simulink model "CM340A_AdcDiagc"  (R2013b)
settings: Solver=FixedStepDiscrete  SolverMode=SingleTasking  StartTime=0.0  StopTime=1  FixedStep=0.002  RelTol=1e-3
values from neighbouring files (symbols this model uses):
  Adc0Diagc = DataDict.NTC    [CM340A_AdcDiagc_DataDict.m]
  Adc1Diagc = DataDict.NTC    [CM340A_AdcDiagc_DataDict.m]
  ADCDIAG0REFVOLT_VOLT_F32 = DataDict.Constant    [CM340A_AdcDiagc_DataDict.m]
  ADCDIAG2REFVOLT_VOLT_F32 = DataDict.Constant    [CM340A_AdcDiagc_DataDict.m]
  ADCDIAG4REFVOLT_VOLT_F32 = DataDict.Constant    [CM340A_AdcDiagc_DataDict.m]
  AdcDiagcNtc0x032FailStep = DataDict.Calibration    [CM340A_AdcDiagc_DataDict.m]
  AdcDiagcNtc0x032PassStep = DataDict.Calibration    [CM340A_AdcDiagc_DataDict.m]
  AdcDiagcNtc0x033FailStep = DataDict.Calibration    [CM340A_AdcDiagc_DataDict.m]
  AdcDiagcNtc0x033PassStep = DataDict.Calibration    [CM340A_AdcDiagc_DataDict.m]
  AdcDiagcSt = DataDict.PIM    [CM340A_AdcDiagc_DataDict.m]
  ADCDIAGPARFLTPRM_CNT_U08 = DataDict.Constant    [CM340A_AdcDiagc_DataDict.m]
  ADCDIAGSCANGROUP2REFFLTPRM_CNT_U08 = DataDict.Constant    [CM340A_AdcDiagc_DataDict.m]
  ADCDIAGSCANGROUP3REFFLTPRM_CNT_U08 = DataDict.Constant    [CM340A_AdcDiagc_DataDict.m]
  ADCDIAGSCANGROUPENDREFVOLT_VOLT_F32 = DataDict.Constant    [CM340A_AdcDiagc_DataDict.m]
  ADCDIAGSCANGROUPSTRTREFVOLT_VOLT_F32 = DataDict.Constant    [CM340A_AdcDiagc_DataDict.m]
  ADCDNECRPARERRCLR_CNT_U08 = DataDict.Constant    [CM340A_AdcDiagc_DataDict.m]
  ADCDNPERPARERRMASK_CNT_U08 = DataDict.Constant    [CM340A_AdcDiagc_DataDict.m]
  VIRTCH21_CNT_U08 = DataDict.Constant    [CM340A_AdcDiagc_DataDict.m]
  VIRTCH22_CNT_U08 = DataDict.Constant    [CM340A_AdcDiagc_DataDict.m]
  VIRTCH23_CNT_U08 = DataDict.Constant    [CM340A_AdcDiagc_DataDict.m]
undefined symbols (not defined in the file or in its folder): NtcSts1, sigbuilder_block, SigQlfr1
libraries: simulink x42, CM340A_AdcDiagc_Library x40
(part 4 of 4)

== system CM340A_AdcDiagc/AdcDiagc/AdcDiagcPer1/NTC Fault Processing1/SetNtcSts/Enabled Subsystem ==
  In1 : Inport
  Enable : EnablePort
  Bitwise Operator : simulink/Logic and Bit Operations/Bitwise Operator  logicop=OR  UseBitMask=off  NumInputPorts=2  BitMask=bin2dec('11011001')  BitMaskRealWorld=Stored Integer
  CopyRight2 : Subsystem  Description=|  mask(Copyright Information){none=on}
      | Copyright info block.                                               
      |                                                                     
      | Place copyright information at the top of every subsystem in design.
      mask prompts: none "No parameters"
      mask help: Place copyright information at the top of every subsystem in design.
      mask Display:
      | NxtrConf = 'Nexteer Confidential';
      | 
      | sys = bdroot; %handle for the current model ("system")
      | first = get_param(sys,'Created');
      | first = first(end-3:end);  %year is last four digits
      | 
      | last = get_param(sys,'LastModifiedDate');
      | if isempty(last)
      |     last = datestr(now,'yyyy');
      | else
      |     last = last(end-3:end);
      | end
      | 
      | if strcmp(first,last)
      |     fprintf('%s -- Copyright %s Nexteer',NxtrConf,first)
      | else
      |     fprintf('%s -- %s%s- %s Nexteer',NxtrConf,char(169),first,last)
      | end
  Data Store Read : DataStoreRead  DataStoreName=Adc1DynDiagcPrm
  Data Store Write1 : DataStoreWrite  DataStoreName=Adc1DynDiagcPrm
  wires:
  In1/1 -> Bitwise Operator/1
  Bitwise Operator/1 -> Data Store Write1/1
  Data Store Read/1 -> Bitwise Operator/2

== system CM340A_AdcDiagc/AdcDiagc/AdcDiagcPer1/Adc Daigc Pointer/Strt & End Ptr Store/State 0/CopyRight2 ==

== system CM340A_AdcDiagc/AdcDiagc/AdcDiagcPer1/Adc Daigc Pointer/Strt & End Ptr Store/State 1/CopyRight2 ==

== system CM340A_AdcDiagc/AdcDiagc/AdcDiagcPer1/Adc Daigc Pointer/Strt & End Ptr Store/State 2/CopyRight2 ==

== system CM340A_AdcDiagc/AdcDiagc/AdcDiagcPer1/Adc Daigc Pointer/Strt & End Ptr Store/State 4/CopyRight2 ==

== system CM340A_AdcDiagc/AdcDiagc/AdcDiagcPer1/Adc Daigc Pointer/Strt & End Ptr Store/State 6/CopyRight2 ==

== system CM340A_AdcDiagc/AdcDiagc/AdcDiagcPer1/Adc0 Diagc/Adc0 Scan Group Strt and End Ref Voltage Diagc/Subsystem/CopyRight2 ==

== system CM340A_AdcDiagc/AdcDiagc/AdcDiagcPer1/Adc0 Diagc/Adc0 Scan Group Strt and End Ref Voltage Diagc/Subsystem1/CopyRight2 ==

== system CM340A_AdcDiagc/AdcDiagc/AdcDiagcPer1/Adc0 Diagc/State 0, 2, 4, 6/State 0/CopyRight2 ==

== system CM340A_AdcDiagc/AdcDiagc/AdcDiagcPer1/Adc0 Diagc/State 0, 2, 4, 6/State 0/Subsystem ==
  Parameter Byte : Inport
  FltCntrPrev : Inport  Port=2
  Add : Sum
  Bitwise Operator : simulink/Logic and Bit Operations/Bitwise Operator  logicop=AND  UseBitMask=off  NumInputPorts=2  BitMask=bin2dec('01111111')  BitMaskRealWorld=Stored Integer
  Constant : Constant  Value=0
  Constant1 : Constant  Value=127  OutDataTypeStr=uint8
  CopyRight2 : Subsystem  Description=|  mask(Copyright Information){none=on}
      | Copyright info block.                                               
      |                                                                     
      | Place copyright information at the top of every subsystem in design.
      mask prompts: none "No parameters"
      mask help: Place copyright information at the top of every subsystem in design.
      mask Display:
      | NxtrConf = 'Nexteer Confidential';
      | 
      | sys = bdroot; %handle for the current model ("system")
      | first = get_param(sys,'Created');
      | first = first(end-3:end);  %year is last four digits
      | 
      | last = get_param(sys,'LastModifiedDate');
      | if isempty(last)
      |     last = datestr(now,'yyyy');
      | else
      |     last = last(end-3:end);
      | end
      | 
      | if strcmp(first,last)
      |     fprintf('%s -- Copyright %s Nexteer',NxtrConf,first)
      | else
      |     fprintf('%s -- %s%s- %s Nexteer',NxtrConf,char(169),first,last)
      | end
  Data Type Conversion2 : DataTypeConversion  OutDataTypeStr=uint8
  Relational Operator : RelationalOperator  Operator=>  OutDataTypeStr=boolean
  Scope1 : Scope  NumInputPorts=2
      settings: ShowLegends=on  TimeRange=1000  YMin=-2~0  YMax=2~256  SaveName=ScopeData3
  FltCntr : Outport
  wires:
  Constant/1 -> Relational Operator/2
  Parameter Byte/1 -> Scope1/1, Relational Operator/1
  Relational Operator/1 -> Data Type Conversion2/1
  Add/1 -> Bitwise Operator/1
  Bitwise Operator/1 -> FltCntr/1, Scope1/2
  FltCntrPrev/1 -> Add/2
  Data Type Conversion2/1 -> Add/1
  Constant1/1 -> Bitwise Operator/2

== system CM340A_AdcDiagc/AdcDiagc/AdcDiagcPer1/Adc0 Diagc/State 0, 2, 4, 6/State 2/CopyRight2 ==

== system CM340A_AdcDiagc/AdcDiagc/AdcDiagcPer1/Adc0 Diagc/State 0, 2, 4, 6/State 2/Subsystem1 ==
  Parameter Byte : Inport
  FltCntrPrev : Inport  Port=2
  Add : Sum
  Bitwise Operator : simulink/Logic and Bit Operations/Bitwise Operator  logicop=AND  UseBitMask=off  NumInputPorts=2  BitMask=bin2dec('01111111')  BitMaskRealWorld=Stored Integer
  Constant : Constant  Value=0
  Constant1 : Constant  Value=127  OutDataTypeStr=uint8
  CopyRight2 : Subsystem  Description=|  mask(Copyright Information){none=on}
      | Copyright info block.                                               
      |                                                                     
      | Place copyright information at the top of every subsystem in design.
      mask prompts: none "No parameters"
      mask help: Place copyright information at the top of every subsystem in design.
      mask Display:
      | NxtrConf = 'Nexteer Confidential';
      | 
      | sys = bdroot; %handle for the current model ("system")
      | first = get_param(sys,'Created');
      | first = first(end-3:end);  %year is last four digits
      | 
      | last = get_param(sys,'LastModifiedDate');
      | if isempty(last)
      |     last = datestr(now,'yyyy');
      | else
      |     last = last(end-3:end);
      | end
      | 
      | if strcmp(first,last)
      |     fprintf('%s -- Copyright %s Nexteer',NxtrConf,first)
      | else
      |     fprintf('%s -- %s%s- %s Nexteer',NxtrConf,char(169),first,last)
      | end
  Data Type Conversion2 : DataTypeConversion  OutDataTypeStr=uint8
  Relational Operator : RelationalOperator  Operator=>  OutDataTypeStr=boolean
  Scope1 : Scope  NumInputPorts=2
      settings: ShowLegends=on  TimeRange=1000  YMin=-2~0  YMax=2~256  SaveName=ScopeData3
  FltCntr : Outport
  wires:
  Constant/1 -> Relational Operator/2
  Parameter Byte/1 -> Scope1/1, Relational Operator/1
  Relational Operator/1 -> Data Type Conversion2/1
  Add/1 -> Bitwise Operator/1
  Bitwise Operator/1 -> FltCntr/1, Scope1/2
  FltCntrPrev/1 -> Add/2
  Data Type Conversion2/1 -> Add/1
  Constant1/1 -> Bitwise Operator/2

== system CM340A_AdcDiagc/AdcDiagc/AdcDiagcPer1/Adc0 Diagc/State 0, 2, 4, 6/State 4/CopyRight2 ==

== system CM340A_AdcDiagc/AdcDiagc/AdcDiagcPer1/Adc0 Diagc/State 0, 2, 4, 6/State 4/Subsystem ==
  Parameter Byte : Inport
  FltCntrPrev : Inport  Port=2
  Add : Sum
  Bitwise Operator : simulink/Logic and Bit Operations/Bitwise Operator  logicop=AND  UseBitMask=off  NumInputPorts=2  BitMask=bin2dec('01111111')  BitMaskRealWorld=Stored Integer
  Constant : Constant  Value=0
  Constant1 : Constant  Value=127  OutDataTypeStr=uint8
  CopyRight2 : Subsystem  Description=|  mask(Copyright Information){none=on}
      | Copyright info block.                                               
      |                                                                     
      | Place copyright information at the top of every subsystem in design.
      mask prompts: none "No parameters"
      mask help: Place copyright information at the top of every subsystem in design.
      mask Display:
      | NxtrConf = 'Nexteer Confidential';
      | 
      | sys = bdroot; %handle for the current model ("system")
      | first = get_param(sys,'Created');
      | first = first(end-3:end);  %year is last four digits
      | 
      | last = get_param(sys,'LastModifiedDate');
      | if isempty(last)
      |     last = datestr(now,'yyyy');
      | else
      |     last = last(end-3:end);
      | end
      | 
      | if strcmp(first,last)
      |     fprintf('%s -- Copyright %s Nexteer',NxtrConf,first)
      | else
      |     fprintf('%s -- %s%s- %s Nexteer',NxtrConf,char(169),first,last)
      | end
  Data Type Conversion2 : DataTypeConversion  OutDataTypeStr=uint8
  Relational Operator : RelationalOperator  Operator=>  OutDataTypeStr=boolean
  Scope1 : Scope  NumInputPorts=2
      settings: ShowLegends=on  TimeRange=1000  YMin=-2~0  YMax=2~256  SaveName=ScopeData3
  FltCntr : Outport
  wires:
  Constant/1 -> Relational Operator/2
  Parameter Byte/1 -> Scope1/1, Relational Operator/1
  Relational Operator/1 -> Data Type Conversion2/1
  Add/1 -> Bitwise Operator/1
  Bitwise Operator/1 -> FltCntr/1, Scope1/2
  FltCntrPrev/1 -> Add/2
  Data Type Conversion2/1 -> Add/1
  Constant1/1 -> Bitwise Operator/2

== system CM340A_AdcDiagc/AdcDiagc/AdcDiagcPer1/Adc0 Diagc/State 0, 2, 4, 6/State 6/CopyRight2 ==

== system CM340A_AdcDiagc/AdcDiagc/AdcDiagcPer1/Adc0 Diagc/State 0, 2, 4, 6/State 6/Subsystem ==
  Parameter Byte : Inport
  FltCntrPrev : Inport  Port=2
  Add : Sum
  Bitwise Operator : simulink/Logic and Bit Operations/Bitwise Operator  logicop=AND  UseBitMask=off  NumInputPorts=2  BitMask=bin2dec('01111111')  BitMaskRealWorld=Stored Integer
  Constant : Constant  Value=0
  Constant1 : Constant  Value=127  OutDataTypeStr=uint8
  CopyRight2 : Subsystem  Description=|  mask(Copyright Information){none=on}
      | Copyright info block.                                               
      |                                                                     
      | Place copyright information at the top of every subsystem in design.
      mask prompts: none "No parameters"
      mask help: Place copyright information at the top of every subsystem in design.
      mask Display:
      | NxtrConf = 'Nexteer Confidential';
      | 
      | sys = bdroot; %handle for the current model ("system")
      | first = get_param(sys,'Created');
      | first = first(end-3:end);  %year is last four digits
      | 
      | last = get_param(sys,'LastModifiedDate');
      | if isempty(last)
      |     last = datestr(now,'yyyy');
      | else
      |     last = last(end-3:end);
      | end
      | 
      | if strcmp(first,last)
      |     fprintf('%s -- Copyright %s Nexteer',NxtrConf,first)
      | else
      |     fprintf('%s -- %s%s- %s Nexteer',NxtrConf,char(169),first,last)
      | end
  Data Type Conversion2 : DataTypeConversion  OutDataTypeStr=uint8
  Relational Operator : RelationalOperator  Operator=>  OutDataTypeStr=boolean
  Scope1 : Scope  NumInputPorts=2
      settings: ShowLegends=on  TimeRange=1000  YMin=-2~0  YMax=2~256  SaveName=ScopeData3
  FltCntr : Outport
  wires:
  Constant/1 -> Relational Operator/2
  Parameter Byte/1 -> Scope1/1, Relational Operator/1
  Relational Operator/1 -> Data Type Conversion2/1
  Add/1 -> Bitwise Operator/1
  Bitwise Operator/1 -> FltCntr/1, Scope1/2
  FltCntrPrev/1 -> Add/2
  Data Type Conversion2/1 -> Add/1
  Constant1/1 -> Bitwise Operator/2

== system CM340A_AdcDiagc/AdcDiagc/AdcDiagcPer1/Adc1 Diagc/Adc1 Scan Group Strt and End Ref Voltage Diagc/Subsystem/CopyRight2 ==

== system CM340A_AdcDiagc/AdcDiagc/AdcDiagcPer1/Adc1 Diagc/Adc1 Scan Group Strt and End Ref Voltage Diagc/Subsystem1/CopyRight2 ==

== system CM340A_AdcDiagc/AdcDiagc/AdcDiagcPer1/Adc1 Diagc/State 0,2,4,6/State 0/CopyRight2 ==

== system CM340A_AdcDiagc/AdcDiagc/AdcDiagcPer1/Adc1 Diagc/State 0,2,4,6/State 0/Subsystem ==
  Parameter Byte : Inport
  FltCntrPrev : Inport  Port=2
  Add : Sum
  Bitwise Operator : simulink/Logic and Bit Operations/Bitwise Operator  logicop=AND  UseBitMask=off  NumInputPorts=2  BitMask=bin2dec('01111111')  BitMaskRealWorld=Stored Integer
  Constant : Constant  Value=0
  Constant1 : Constant  Value=127  OutDataTypeStr=uint8
  CopyRight2 : Subsystem  Description=|  mask(Copyright Information){none=on}
      | Copyright info block.                                               
      |                                                                     
      | Place copyright information at the top of every subsystem in design.
      mask prompts: none "No parameters"
      mask help: Place copyright information at the top of every subsystem in design.
      mask Display:
      | NxtrConf = 'Nexteer Confidential';
      | 
      | sys = bdroot; %handle for the current model ("system")
      | first = get_param(sys,'Created');
      | first = first(end-3:end);  %year is last four digits
      | 
      | last = get_param(sys,'LastModifiedDate');
      | if isempty(last)
      |     last = datestr(now,'yyyy');
      | else
      |     last = last(end-3:end);
      | end
      | 
      | if strcmp(first,last)
      |     fprintf('%s -- Copyright %s Nexteer',NxtrConf,first)
      | else
      |     fprintf('%s -- %s%s- %s Nexteer',NxtrConf,char(169),first,last)
      | end
  Data Type Conversion2 : DataTypeConversion  OutDataTypeStr=uint8
  Relational Operator : RelationalOperator  Operator=>  OutDataTypeStr=boolean
  Scope1 : Scope  NumInputPorts=2
      settings: ShowLegends=on  TimeRange=1000  YMin=-2~0  YMax=2~256  SaveName=ScopeData3
  FltCntr : Outport
  wires:
  Constant/1 -> Relational Operator/2
  Parameter Byte/1 -> Scope1/1, Relational Operator/1
  Relational Operator/1 -> Data Type Conversion2/1
  Add/1 -> Bitwise Operator/1
  Bitwise Operator/1 -> FltCntr/1, Scope1/2
  FltCntrPrev/1 -> Add/2
  Data Type Conversion2/1 -> Add/1
  Constant1/1 -> Bitwise Operator/2

== system CM340A_AdcDiagc/AdcDiagc/AdcDiagcPer1/Adc1 Diagc/State 0,2,4,6/State 2/CopyRight2 ==

== system CM340A_AdcDiagc/AdcDiagc/AdcDiagcPer1/Adc1 Diagc/State 0,2,4,6/State 2/Subsystem ==
  Parameter Byte : Inport
  FltCntrPrev : Inport  Port=2
  Add : Sum
  Bitwise Operator : simulink/Logic and Bit Operations/Bitwise Operator  logicop=AND  UseBitMask=off  NumInputPorts=2  BitMask=bin2dec('01111111')  BitMaskRealWorld=Stored Integer
  Constant : Constant  Value=0
  Constant1 : Constant  Value=127  OutDataTypeStr=uint8
  CopyRight2 : Subsystem  Description=|  mask(Copyright Information){none=on}
      | Copyright info block.                                               
      |                                                                     
      | Place copyright information at the top of every subsystem in design.
      mask prompts: none "No parameters"
      mask help: Place copyright information at the top of every subsystem in design.
      mask Display:
      | NxtrConf = 'Nexteer Confidential';
      | 
      | sys = bdroot; %handle for the current model ("system")
      | first = get_param(sys,'Created');
      | first = first(end-3:end);  %year is last four digits
      | 
      | last = get_param(sys,'LastModifiedDate');
      | if isempty(last)
      |     last = datestr(now,'yyyy');
      | else
      |     last = last(end-3:end);
      | end
      | 
      | if strcmp(first,last)
      |     fprintf('%s -- Copyright %s Nexteer',NxtrConf,first)
      | else
      |     fprintf('%s -- %s%s- %s Nexteer',NxtrConf,char(169),first,last)
      | end
  Data Type Conversion2 : DataTypeConversion  OutDataTypeStr=uint8
  Relational Operator : RelationalOperator  Operator=>  OutDataTypeStr=boolean
  Scope1 : Scope  NumInputPorts=2
      settings: ShowLegends=on  TimeRange=1000  YMin=-2~0  YMax=2~256  SaveName=ScopeData3
  FltCntr : Outport
  wires:
  Constant/1 -> Relational Operator/2
  Parameter Byte/1 -> Scope1/1, Relational Operator/1
  Relational Operator/1 -> Data Type Conversion2/1
  Add/1 -> Bitwise Operator/1
  Bitwise Operator/1 -> FltCntr/1, Scope1/2
  FltCntrPrev/1 -> Add/2
  Data Type Conversion2/1 -> Add/1
  Constant1/1 -> Bitwise Operator/2

== system CM340A_AdcDiagc/AdcDiagc/AdcDiagcPer1/Adc1 Diagc/State 0,2,4,6/State 4/CopyRight2 ==

== system CM340A_AdcDiagc/AdcDiagc/AdcDiagcPer1/Adc1 Diagc/State 0,2,4,6/State 4/Subsystem ==
  Parameter Byte : Inport
  FltCntrPrev : Inport  Port=2
  Add : Sum
  Bitwise Operator : simulink/Logic and Bit Operations/Bitwise Operator  logicop=AND  UseBitMask=off  NumInputPorts=2  BitMask=bin2dec('01111111')  BitMaskRealWorld=Stored Integer
  Constant : Constant  Value=0
  Constant1 : Constant  Value=127  OutDataTypeStr=uint8
  CopyRight2 : Subsystem  Description=|  mask(Copyright Information){none=on}
      | Copyright info block.                                               
      |                                                                     
      | Place copyright information at the top of every subsystem in design.
      mask prompts: none "No parameters"
      mask help: Place copyright information at the top of every subsystem in design.
      mask Display:
      | NxtrConf = 'Nexteer Confidential';
      | 
      | sys = bdroot; %handle for the current model ("system")
      | first = get_param(sys,'Created');
      | first = first(end-3:end);  %year is last four digits
      | 
      | last = get_param(sys,'LastModifiedDate');
      | if isempty(last)
      |     last = datestr(now,'yyyy');
      | else
      |     last = last(end-3:end);
      | end
      | 
      | if strcmp(first,last)
      |     fprintf('%s -- Copyright %s Nexteer',NxtrConf,first)
      | else
      |     fprintf('%s -- %s%s- %s Nexteer',NxtrConf,char(169),first,last)
      | end
  Data Type Conversion2 : DataTypeConversion  OutDataTypeStr=uint8
  Relational Operator : RelationalOperator  Operator=>  OutDataTypeStr=boolean
  Scope1 : Scope  NumInputPorts=2
      settings: ShowLegends=on  TimeRange=1000  YMin=-2~0  YMax=2~256  SaveName=ScopeData3
  FltCntr : Outport
  wires:
  Constant/1 -> Relational Operator/2
  Parameter Byte/1 -> Scope1/1, Relational Operator/1
  Relational Operator/1 -> Data Type Conversion2/1
  Add/1 -> Bitwise Operator/1
  Bitwise Operator/1 -> FltCntr/1, Scope1/2
  FltCntrPrev/1 -> Add/2
  Data Type Conversion2/1 -> Add/1
  Constant1/1 -> Bitwise Operator/2

== system CM340A_AdcDiagc/AdcDiagc/AdcDiagcPer1/Adc1 Diagc/State 0,2,4,6/State 6/CopyRight2 ==

== system CM340A_AdcDiagc/AdcDiagc/AdcDiagcPer1/Adc1 Diagc/State 0,2,4,6/State 6/Subsystem ==
  Parameter Byte : Inport
  FltCntrPrev : Inport  Port=2
  Add : Sum
  Bitwise Operator : simulink/Logic and Bit Operations/Bitwise Operator  logicop=AND  UseBitMask=off  NumInputPorts=2  BitMask=bin2dec('01111111')  BitMaskRealWorld=Stored Integer
  Constant : Constant  Value=0
  Constant1 : Constant  Value=127  OutDataTypeStr=uint8
  CopyRight2 : Subsystem  Description=|  mask(Copyright Information){none=on}
      | Copyright info block.                                               
      |                                                                     
      | Place copyright information at the top of every subsystem in design.
      mask prompts: none "No parameters"
      mask help: Place copyright information at the top of every subsystem in design.
      mask Display:
      | NxtrConf = 'Nexteer Confidential';
      | 
      | sys = bdroot; %handle for the current model ("system")
      | first = get_param(sys,'Created');
      | first = first(end-3:end);  %year is last four digits
      | 
      | last = get_param(sys,'LastModifiedDate');
      | if isempty(last)
      |     last = datestr(now,'yyyy');
      | else
      |     last = last(end-3:end);
      | end
      | 
      | if strcmp(first,last)
      |     fprintf('%s -- Copyright %s Nexteer',NxtrConf,first)
      | else
      |     fprintf('%s -- %s%s- %s Nexteer',NxtrConf,char(169),first,last)
      | end
  Data Type Conversion2 : DataTypeConversion  OutDataTypeStr=uint8
  Relational Operator : RelationalOperator  Operator=>  OutDataTypeStr=boolean
  Scope1 : Scope  NumInputPorts=2
      settings: ShowLegends=on  TimeRange=1000  YMin=-2~0  YMax=2~256  SaveName=ScopeData3
  FltCntr : Outport
  wires:
  Constant/1 -> Relational Operator/2
  Parameter Byte/1 -> Scope1/1, Relational Operator/1
  Relational Operator/1 -> Data Type Conversion2/1
  Add/1 -> Bitwise Operator/1
  Bitwise Operator/1 -> FltCntr/1, Scope1/2
  FltCntrPrev/1 -> Add/2
  Data Type Conversion2/1 -> Add/1
  Constant1/1 -> Bitwise Operator/2

== system CM340A_AdcDiagc/AdcDiagc/AdcDiagcPer1/NTC Fault Processing0/Atomic Subsystem/Fail Step/CopyRight2 ==

== system CM340A_AdcDiagc/AdcDiagc/AdcDiagcPer1/NTC Fault Processing0/Atomic Subsystem/Pass Step/CopyRight2 ==

== system CM340A_AdcDiagc/AdcDiagc/AdcDiagcPer1/NTC Fault Processing0/SetNtcSts/Enabled Subsystem/CopyRight2 ==

== system CM340A_AdcDiagc/AdcDiagc/AdcDiagcPer1/NTC Fault Processing1/Atomic Subsystem/Fail Step/CopyRight2 ==

== system CM340A_AdcDiagc/AdcDiagc/AdcDiagcPer1/NTC Fault Processing1/Atomic Subsystem/Pass Step/CopyRight2 ==

== system CM340A_AdcDiagc/AdcDiagc/AdcDiagcPer1/NTC Fault Processing1/SetNtcSts/Enabled Subsystem/CopyRight2 ==

== system CM340A_AdcDiagc/AdcDiagc/AdcDiagcPer1/Adc0 Diagc/State 0, 2, 4, 6/State 0/Subsystem/CopyRight2 ==

== system CM340A_AdcDiagc/AdcDiagc/AdcDiagcPer1/Adc0 Diagc/State 0, 2, 4, 6/State 2/Subsystem1/CopyRight2 ==

== system CM340A_AdcDiagc/AdcDiagc/AdcDiagcPer1/Adc0 Diagc/State 0, 2, 4, 6/State 4/Subsystem/CopyRight2 ==

== system CM340A_AdcDiagc/AdcDiagc/AdcDiagcPer1/Adc0 Diagc/State 0, 2, 4, 6/State 6/Subsystem/CopyRight2 ==

== system CM340A_AdcDiagc/AdcDiagc/AdcDiagcPer1/Adc1 Diagc/State 0,2,4,6/State 0/Subsystem/CopyRight2 ==

== system CM340A_AdcDiagc/AdcDiagc/AdcDiagcPer1/Adc1 Diagc/State 0,2,4,6/State 2/Subsystem/CopyRight2 ==

== system CM340A_AdcDiagc/AdcDiagc/AdcDiagcPer1/Adc1 Diagc/State 0,2,4,6/State 4/Subsystem/CopyRight2 ==

== system CM340A_AdcDiagc/AdcDiagc/AdcDiagcPer1/Adc1 Diagc/State 0,2,4,6/State 6/Subsystem/CopyRight2 ==

== stateflow chart CM340A_AdcDiagc/AdcDiagc/AdcDiagcPer1/NTC Fault Processing1/SetNtcSts/ISO Fault Debounce Design ==
  note: NTCSTS_PASSD           (0)
      | NTCSTS_FAILD             (1)
      | NTCSTS_PREPASSD   (2)
      | NTCSTS_PREFAILD     (3)
      |
      | SIGQLFR_NORES        (0)
      | SIGQLFR_PASSD         (1)
      | SIGQLFR_FAILD           (2)
  note: Pass Loop
  note: Fail Loop
  note: 
  (default) -> (junction 89)
  (junction 89) -> (junction 95) [order 1] : [NtcSts ==3]
  (junction 89) -> (junction 93) [order 2] : [NtcSts ==2]
  (junction 89) -> (junction 141) [order 3] : [NtcSts ==1]
      | { ErrAcc = 32767;
      | Qualifier =2;
      |  }
  (junction 89) -> (junction 141) [order 4] : [NtcSts ==0]
      | { ErrAcc = -32768;
      | Qualifier=1;
      | }
  (junction 95) -> (junction 103) [order 2]
  (junction 95) -> (junction 111) [order 1] : [ErrAcc <=0]
      | {ErrAcc = DebStep;}
  (junction 93) -> (junction 123) [order 2] : {
      | ErrAcc = ErrAcc - DebStep;
      | }
  (junction 93) -> (junction 123) [order 1] : [(ErrAcc - DebStep) <= -32768]
      | { ErrAcc = -32768;
      | Qualifier=1;
      | }
  (junction 103) -> (junction 111) [order 1] : [(ErrAcc + DebStep) <32767]
      | {ErrAcc = ErrAcc + DebStep;}
  (junction 103) -> (junction 111) [order 2] : {ErrAcc = 32767;
      | Qualifier =2;}
  (junction 123) -> (junction 141)
  (junction 111) -> (junction 141)
  (junction 141) -> (junction 159) [order 2] : {ErrAcc = 0;
      | Qualifier =0;
      | }
  (junction 141) -> (junction 159) [order 1] : [SvcClr ==0]
  (junction 159) -> (junction 212) : {
      | ErrAccOut = ErrAcc;
      | }
  data: NtcSts input uint8; Qualifier output uint8; DebStep input uint16; ErrAcc local int16; SvcClr input; ErrAccOut output int16

== stateflow chart CM340A_AdcDiagc/AdcDiagc/AdcDiagcPer1/NTC Fault Processing0/SetNtcSts/ISO Fault Debounce Design ==
  note: NTCSTS_PASSD           (0)
      | NTCSTS_FAILD             (1)
      | NTCSTS_PREPASSD   (2)
      | NTCSTS_PREFAILD     (3)
      |
      | SIGQLFR_NORES        (0)
      | SIGQLFR_PASSD         (1)
      | SIGQLFR_FAILD           (2)
  note: Pass Loop
  note: Fail Loop
  note: 
  (default) -> (junction 238)
  (junction 238) -> (junction 236) [order 1] : [NtcSts ==3]
  (junction 238) -> (junction 241) [order 2] : [NtcSts ==2]
  (junction 238) -> (junction 233) [order 3] : [NtcSts ==1]
      | { ErrAcc = 32767;
      | Qualifier =2;
      |  }
  (junction 238) -> (junction 233) [order 4] : [NtcSts ==0]
      | { ErrAcc = -32768;
      | Qualifier=1;
      | }
  (junction 236) -> (junction 235) [order 2]
  (junction 236) -> (junction 237) [order 1] : [ErrAcc <=0]
      | {ErrAcc = DebStep;}
  (junction 241) -> (junction 234) [order 2] : {
      | ErrAcc = ErrAcc - DebStep;
      | }
  (junction 241) -> (junction 234) [order 1] : [(ErrAcc - DebStep) <= -32768]
      | { ErrAcc = -32768;
      | Qualifier=1;
      | }
  (junction 235) -> (junction 237) [order 1] : [(ErrAcc + DebStep) <32767]
      | {ErrAcc = ErrAcc + DebStep;}
  (junction 235) -> (junction 237) [order 2] : {ErrAcc = 32767;
      | Qualifier =2;}
  (junction 234) -> (junction 233)
  (junction 237) -> (junction 233)
  (junction 233) -> (junction 232) [order 2] : {ErrAcc = 0;
      | Qualifier =0;
      | }
  (junction 233) -> (junction 232) [order 1] : [SvcClr ==0]
  (junction 232) -> (junction 231) : {
      | ErrAccOut = ErrAcc;
      | }
  data: NtcSts input uint8; Qualifier output uint8; DebStep input uint16; ErrAcc local int16; SvcClr input; ErrAccOut output int16
